simulink model "SIGAS_SensorModel"  (R2026a)
settings: Solver=FixedStepDiscrete  StopTime=Test_DefaultStopTime  FixedStep=Timing_PressureSample
undefined symbols (not defined in the file): GasSensor_AdcMax, GasSensor_AdcMin, GasSensor_ResponseTau, Timing_GasSample
settings Model: DataDictionary=sigas_rt.sldd  Creator=josue  LastModifiedBy=josue

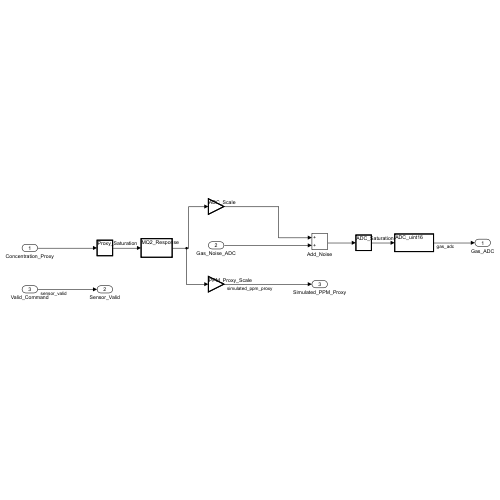
[thumbnail: Simulink's stored preview of the top-level diagram]
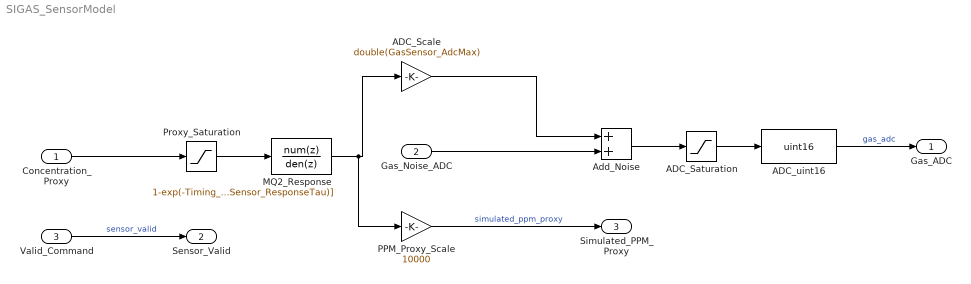
== system SIGAS_SensorModel ==
  Concentration_Proxy : Inport  OutDataTypeStr=double  PortDimensions=3  SampleTime=0.1
  Gas_Noise_ADC : Inport  Port=2  OutDataTypeStr=double  PortDimensions=3  SampleTime=0.1
  Valid_Command : Inport  Port=3  OutDataTypeStr=boolean  PortDimensions=3  SampleTime=0.05
  ADC_Saturation : Saturate  UpperLimit=double(GasSensor_AdcMax)  LowerLimit=double(GasSensor_AdcMin)
  ADC_Scale : Gain  Gain=double(GasSensor_AdcMax)
  ADC_uint16 : DataTypeConversion  OutDataTypeStr=uint16  SaturateOnIntegerOverflow=off  RndMeth=Floor
  Add_Noise : Sum
  MQ2_Response : DiscreteTransferFcn  Numerator=1-exp(-Timing_GasSample/GasSensor_ResponseTau)  Denominator=[1 -exp(-Timing_GasSample/GasSensor_ResponseTau)]  SampleTime=Timing_GasSample
  PPM_Proxy_Scale : Gain  Gain=10000
  Proxy_Saturation : Saturate  UpperLimit=1  LowerLimit=0
  Gas_ADC : Outport
  Sensor_Valid : Outport  Port=2
  Simulated_PPM_Proxy : Outport  Port=3
  wires:
  PPM_Proxy_Scale/1 -> Simulated_PPM_Proxy/1  "simulated_ppm_proxy"
  Valid_Command/1 -> Sensor_Valid/1  "sensor_valid"
  ADC_uint16/1 -> Gas_ADC/1  "gas_adc"
  ADC_Saturation/1 -> ADC_uint16/1
  Add_Noise/1 -> ADC_Saturation/1
  Gas_Noise_ADC/1 -> Add_Noise/2
  ADC_Scale/1 -> Add_Noise/1
  MQ2_Response/1 -> ADC_Scale/1, PPM_Proxy_Scale/1
  Proxy_Saturation/1 -> MQ2_Response/1
  Concentration_Proxy/1 -> Proxy_Saturation/1
